simulink model "BaseEngineController_LS_128"  (Simulink 7.7)
settings: Solver=FixedStepDiscrete  StartTime=0.0  StopTime=10.0  RelTol=1e-3
PreLoadFcn:
  | try, eval([bdroot '_setup']); catch, eval('model_setup', ''); end
InitFcn:
  | try, eval([bdroot '_setup']); catch, eval('model_setup', ''); end
undefined symbols (not defined in the file): ECU565, High, motohawk_build_version, motohawk_trunc_name, motohawk_vardec_config_group, motohawk_vardec_path, True
libraries: MotoHawk_lib x1418, motohawk_control_primitives_lib x183, motohawk_engine_lib x32, simulink x21, motohawk_annotations_lib x9, AutoDoc_lib x8, simulink_extras x4, motohawk_ccp_examples_lib x1, motohawk_control_primitives_motoshare_lib x1
(part 9 of 27)

== system BaseEngineController_LS_128/Foreground/Inputs/NonLinearSensors/Temp Sensors ==
  Trigger : TriggerPort  TriggerType=function-call
  CAT1 : motohawk_engine_lib/Non-Linear Sensor Characterization (tbl)  SystemSampleTime=-1  nam='CAT'  prefix='CAT'  units='C'  inputunits='ADC'  parent_group=motohawk_vardec_path(gcb)  tblsize=13  samp_time=-1
  "ECT " : motohawk_engine_lib/Non-Linear Sensor Characterization (tbl)  SystemSampleTime=-1  nam='ECT'  prefix='ECT'  units='C'  inputunits='ADC'  parent_group=motohawk_vardec_path(gcb)  tblsize=13  samp_time=-1
  "EVAP " : motohawk_engine_lib/Non-Linear Sensor Characterization (tbl)  SystemSampleTime=-1  nam='EVAP'  prefix='EVAP'  units='C'  inputunits='ADC'  parent_group=motohawk_vardec_path(gcb)  tblsize=13  samp_time=-1
  "IAT " : motohawk_engine_lib/Non-Linear Sensor Characterization (tbl)  SystemSampleTime=-1  nam='IAT'  prefix='IAT'  units='C'  inputunits='ADC'  parent_group=motohawk_vardec_path(gcb)  tblsize=13  samp_time=-1
  motohawk_ain : MotoHawk_lib/Analog I//O Blocks/motohawk_ain  res_name=[]  text_resource=AN10M  code_resource=RES_ECUP  val_resource=-1  target=ECU565-128  resource_enum_str=(None)=-1,ECUP=53,DRVP=54,XDRP=55,AN1M=56,AN2M=57,AN3M=58,AN4M=59,AN5M=60,AN6M=61,AN7M=62,AN8M=63,AN9M=64,AN10M=65,AN11M=66,AN12M=67,AN13M=68,AN14M=69,AN15M=70,AN16M=71,AN17M=72,AN18M=73,AN19M=74,AN20M=75,AN21M=76,AN22M=77,AN23M=78,AN24M=79,AN25M=80,AN26M=81,AN27M=82,AN28M=83,AN29M=84,AN30M=85,AN31M=86,AN32M=87,AN33M=88,AN34M=89,O2A=90,O2B=91,XDRP_B=92,REF_14V=143  altref=5V Reference  typ=uint16  num_adc_bits=10  use_stat=off  use_vardec=on  nam='ECTSensorPin'  read_level=1  write_level=1  group='System | I/O Pins | Inputs Config'
  motohawk_ain1 : MotoHawk_lib/Analog I//O Blocks/motohawk_ain  res_name=[]  text_resource=AN9M  code_resource=RES_ECUP  val_resource=-1  target=ECU565-128  resource_enum_str=(None)=-1,ECUP=53,DRVP=54,XDRP=55,AN1M=56,AN2M=57,AN3M=58,AN4M=59,AN5M=60,AN6M=61,AN7M=62,AN8M=63,AN9M=64,AN10M=65,AN11M=66,AN12M=67,AN13M=68,AN14M=69,AN15M=70,AN16M=71,AN17M=72,AN18M=73,AN19M=74,AN20M=75,AN21M=76,AN22M=77,AN23M=78,AN24M=79,AN25M=80,AN26M=81,AN27M=82,AN28M=83,AN29M=84,AN30M=85,AN31M=86,AN32M=87,AN33M=88,AN34M=89,O2A=90,O2B=91,XDRP_B=92,REF_14V=143  altref=5V Reference  typ=uint16  num_adc_bits=10  use_stat=off  use_vardec=on  nam='IATSensorPin'  read_level=1  write_level=1  group='System | I/O Pins | Inputs Config'
  motohawk_ain2 : MotoHawk_lib/Analog I//O Blocks/motohawk_ain  res_name=[]  text_resource=AN11M  code_resource=RES_ECUP  val_resource=-1  target=ECU565-128  resource_enum_str=(None)=-1,ECUP=53,DRVP=54,XDRP=55,AN1M=56,AN2M=57,AN3M=58,AN4M=59,AN5M=60,AN6M=61,AN7M=62,AN8M=63,AN9M=64,AN10M=65,AN11M=66,AN12M=67,AN13M=68,AN14M=69,AN15M=70,AN16M=71,AN17M=72,AN18M=73,AN19M=74,AN20M=75,AN21M=76,AN22M=77,AN23M=78,AN24M=79,AN25M=80,AN26M=81,AN27M=82,AN28M=83,AN29M=84,AN30M=85,AN31M=86,AN32M=87,AN33M=88,AN34M=89,O2A=90,O2B=91,XDRP_B=92,REF_14V=143  altref=5V Reference  typ=uint16  num_adc_bits=10  use_stat=off  use_vardec=on  nam='EVAPSensorPin'  read_level=1  write_level=1  group='System | I/O Pins | Inputs Config'
  motohawk_ain3 : MotoHawk_lib/Analog I//O Blocks/motohawk_ain  res_name=[]  text_resource=AN12M  code_resource=RES_ECUP  val_resource=-1  target=ECU565-128  resource_enum_str=(None)=-1,ECUP=53,DRVP=54,XDRP=55,AN1M=56,AN2M=57,AN3M=58,AN4M=59,AN5M=60,AN6M=61,AN7M=62,AN8M=63,AN9M=64,AN10M=65,AN11M=66,AN12M=67,AN13M=68,AN14M=69,AN15M=70,AN16M=71,AN17M=72,AN18M=73,AN19M=74,AN20M=75,AN21M=76,AN22M=77,AN23M=78,AN24M=79,AN25M=80,AN26M=81,AN27M=82,AN28M=83,AN29M=84,AN30M=85,AN31M=86,AN32M=87,AN33M=88,AN34M=89,O2A=90,O2B=91,XDRP_B=92,REF_14V=143  altref=5V Reference  typ=uint16  num_adc_bits=10  use_stat=off  use_vardec=on  nam='CATSensorPin'  read_level=1  write_level=1  group='System | I/O Pins | Inputs Config'
  ECT : Outport
  ECT_Raw : Outport  Port=2
  IAT : Outport  Port=3
  IAT_Raw : Outport  Port=4
  EVAP : Outport  Port=5
  EVAP_Raw : Outport  Port=6
  CAT : Outport  Port=7
  CAT_Raw : Outport  Port=8
  wires:
  motohawk_ain1/1 -> "IAT "/1
  motohawk_ain/1 -> "ECT "/1
  "ECT "/1 -> ECT/1
  "ECT "/2 -> ECT_Raw/1
  "IAT "/1 -> IAT/1  "IAT"
  "IAT "/2 -> IAT_Raw/1  "IAT_Raw"
  motohawk_ain2/1 -> "EVAP "/1
  "EVAP "/1 -> EVAP/1  "IAT"
  "EVAP "/2 -> EVAP_Raw/1  "IAT_Raw"
  motohawk_ain3/1 -> CAT1/1
  CAT1/1 -> CAT/1  "IAT"
  CAT1/2 -> CAT_Raw/1  "IAT_Raw"

== system BaseEngineController_LS_128/Foreground/Inputs/PotentiometerSensors/APP1 ==
  note: Non-Linear Scaling from ADC Counts
      | to Engineering Units
  note: Faults for
      | Out-of-Range
      | Input
  ADC : Inport
  Constant1 : Constant  Value=0  OutDataTypeStr=double
  Data Type Conversion : DataTypeConversion  SaturateOnIntegerOverflow=on  RndMeth=Zero
  Final Value : MotoHawk_lib/Calibration & Probing Blocks/motohawk_probe  nam=nam  show_more=on  name_source=Use Parameter  read_level=1  view_as=Number  enum_struct={'Disabled', 'Enabled'}  vector_style=Wide Row  use_help_units=on  help='Final value after Linear Sensor Characterization'  units=units  use_header_enum=off  row_header_enum={}  col_header_enum={}  use_precision=off  precision=''  gain=1  offset=0  exp=1  use_mototune_group=on  mototune_group=group
  First Order Low Pass : motohawk_control_primitives_lib/First Order Low Pass (Tunable)  SystemSampleTime=-1  nam=[prefix 'FiltConst']  samp_time=samp_time  group=[group ' | ' nam ' Config']
  From Analog Input : MotoHawk_lib/Calibration & Probing Blocks/motohawk_probe  nam=[prefix 'ADC']  show_more=on  name_source=Use Parameter  read_level=1  view_as=Number  enum_struct={'Disabled', 'Enabled'}  vector_style=Wide Row  use_help_units=on  help='Signal measured directly from sensor'  units=inputunits  use_header_enum=off  row_header_enum={}  col_header_enum={}  use_precision=off  precision=''  gain=1  offset=0  exp=1  use_mototune_group=on  mototune_group=group
  If : If  NumInputs=2  IfExpression=u1  ElseIfExpressions=u2  ZeroCross=off
  If Action Subsystem : Subsystem  TreatAsAtomicUnit=on
      mask Display: disp('Saturate');
  If Action Subsystem1 : Subsystem  TreatAsAtomicUnit=on
      mask Display: disp('Default');
  If Action Subsystem2 : Subsystem  TreatAsAtomicUnit=on
      mask Display: disp('Pass Through');
  Logical Operator1 : Logic  Operator=OR
  Logical Operator2 : Logic
  Logical Operator3 : Logic
  Logical Operator4 : Logic  Operator=OR
  Logical Operator5 : Logic
  Logical Operator6 : Logic  Operator=NOT
  Merge : Merge  Inputs=3
  Override : MotoHawk_lib/Calibration & Probing Blocks/motohawk_override_abs  SystemSampleTime=-1  parent_name=nam  parent_val=0  show_more=on  name_source=Use Parameter  parent_read_level=1  parent_override_level=1  view_as=Number  enum_struct={'Disabled', 'Enabled'}  use_help_units=on  parent_help='Override result of linear sensor characterization, in engineering units'  parent_units=units  use_min_max=on  parent_min=-inf  parent_max=inf  use_precision=off  parent_precision=''  parent_gain=1  parent_offset=0  parent_exp=1  use_mototune_group=on  parent_group=group
  Relational Operator2 : RelationalOperator  Operator=>  ZeroCross=off  InputSameDT=on
  Relational Operator3 : RelationalOperator  Operator=<  ZeroCross=off  InputSameDT=on
  Saturation : motohawk_control_primitives_lib/Saturation  SystemSampleTime=-1
  "Unfiltered, Before Range Checking" : MotoHawk_lib/Calibration & Probing Blocks/motohawk_probe  nam=[prefix 'Raw']  show_more=on  name_source=Use Parameter  read_level=1  view_as=Number  enum_struct={'Disabled', 'Enabled'}  vector_style=Wide Row  use_help_units=on  help='After conversion to engineering units, before range checking'  units=units  use_header_enum=off  row_header_enum={}  col_header_enum={}  use_precision=off  precision=''  gain=1  offset=0  exp=1  use_mototune_group=on  mototune_group=group
  Unit Delay : UnitDelay  SampleTime=-1
  motohawk_calibration1 : MotoHawk_lib/Calibration & Probing Blocks/motohawk_calibration  nam=[prefix 'Max']  val=1020  storage=Calibration  show_more=on  name_source=Use Parameter  data_type=double  read_level=1  write_level=1  ovr_cals=on  view_as=Number  enum_struct={'Disabled', 'Enabled'}  vector_style=Wide Row  use_help_units=on  help='Maximum allowable input, indicating short or open circuit'  units=inputunits  use_header_enum=off  row_header_enum={}  col_header_enum={}  use_min_max=off  min_val=-inf  max_val=inf  use_precision=off  precision=''  gain=1  offset=0  exp=1  use_mototune_group=on  mototune_group=[group ' | ' nam ' Config']
  motohawk_calibration2 : MotoHawk_lib/Calibration & Probing Blocks/motohawk_calibration  nam=[prefix 'MaxLimit']  val=100  storage=Calibration  show_more=on  name_source=Use Parameter  data_type=double  read_level=1  write_level=1  ovr_cals=on  view_as=Number  enum_struct={'Disabled', 'Enabled'}  vector_style=Wide Row  use_help_units=on  help='Sets the upper limit on the potentiometer range.'  units=units  use_header_enum=off  row_header_enum={}  col_header_enum={}  use_min_max=off  min_val=-inf  max_val=inf  use_precision=off  precision=''  gain=1  offset=0  exp=1  use_mototune_group=on  mototune_group=[group ' | ' nam ' Config']
  motohawk_calibration3 : MotoHawk_lib/Calibration & Probing Blocks/motohawk_calibration  nam=[prefix 'Default']  val=0  storage=Calibration  show_more=on  name_source=Use Parameter  data_type=double  read_level=1  write_level=1  ovr_cals=on  view_as=Number  enum_struct={'Disabled', 'Enabled'}  vector_style=Wide Row  use_help_units=on  help="'This is the initial default value should the sensor be in fault on key-up.  Otherwise the sensors outputs the last value prior to faulting'"  units=units  use_header_enum=off  row_header_enum={}  col_header_enum={}  use_min_max=off  min_val=-inf  max_val=inf  use_precision=off  precision=''  gain=1  offset=0  exp=1  use_mototune_group=on  mototune_group=[group ' | ' nam ' Config']
  motohawk_calibration6 : MotoHawk_lib/Calibration & Probing Blocks/motohawk_calibration  nam=[prefix 'Min']  val=10  storage=Calibration  show_more=on  name_source=Use Parameter  data_type=double  read_level=1  write_level=1  ovr_cals=on  view_as=Number  enum_struct={'Disabled', 'Enabled'}  vector_style=Wide Row  use_help_units=on  help='Minimum allowable input, indicating short or open circuit'  units=inputunits  use_header_enum=off  row_header_enum={}  col_header_enum={}  use_min_max=off  min_val=-inf  max_val=inf  use_precision=off  precision=''  gain=1  offset=0  exp=1  use_mototune_group=on  mototune_group=[group ' | ' nam ' Config']
  motohawk_data_read1 : MotoHawk_lib/Data Storage Blocks/motohawk_data_read  source=Lookup By Name  structure=Scalar  operation=Read entire data structure at once  sz_vec=4  sz_row=2  sz_col=3  typ=boolean  nam='MPRD'  checkNull=on  struct_inst_name='Struct1'  struct_nam='MyStruct'
  motohawk_fault_def2 : MotoHawk_lib/Fault Management Blocks/motohawk_fault_def  nam=[prefix 'RangeHigh']  mode=Enabled  id=[]  x=25  y=50  input_suspected=on  indeterminate=off  increment_xy=on  downsample_count=1  ovr_cals=on  ovr_actions=on  show_actions=off  action1_name=''  action1_cond=(None)  action2_name=''  action2_cond=(None)  action3_name=''  action3_cond=(None)  action4_name=''  action4_cond=(None)
  motohawk_fault_def3 : MotoHawk_lib/Fault Management Blocks/motohawk_fault_def  nam=[prefix 'RangeLow']  mode=Enabled  id=[]  x=25  y=50  input_suspected=on  indeterminate=off  increment_xy=on  downsample_count=1  ovr_cals=on  ovr_actions=on  show_actions=off  action1_name=''  action1_cond=(None)  action2_name=''  action2_cond=(None)  action3_name=''  action3_cond=(None)  action4_name=''  action4_cond=(None)
  motohawk_fault_status1 : MotoHawk_lib/Fault Management Blocks/motohawk_fault_status  source=Lookup By Name  nam=[prefix 'RangeHigh']  status=Active
  motohawk_fault_status2 : MotoHawk_lib/Fault Management Blocks/motohawk_fault_status  source=Lookup By Name  nam=[prefix 'RangeHigh']  status=Suspected
  motohawk_fault_status3 : MotoHawk_lib/Fault Management Blocks/motohawk_fault_status  source=Lookup By Name  nam=[prefix 'RangeLow']  status=Suspected
  motohawk_fault_status4 : MotoHawk_lib/Fault Management Blocks/motohawk_fault_status  source=Lookup By Name  nam=[prefix 'RangeLow']  status=Active
  motohawk_table_1d1 : MotoHawk_lib/Lookup Tables/motohawk_table_1d  SystemSampleTime=-1  nam=nam  bp_nam=''  breakpoint_data=[1:tblsize]  table_data=[1:tblsize]  show_more=on  bp_data_type=Inherit from 'Breakpoint Data'  bp_storage=Constant  table_data_type=Inherit from 'Table Data'  storage=NonAdaptive  read_level=1  write_level=1  ovr_cals=on  use_help=on  help='Look up table to allownon-linear characterization of sensors'  bp_units=inputunits  table_units=units  use_min_max=off  bp_min_val=-inf  bp_max_val=inf  min_val=-inf  max_val=inf  use_precision=off  use_breakpoint=off  b_precision=''  b_gain=1  b_offset=0  b_exp=1  use_table=off  t_precision=''  t_gain=1  t_offset=0  t_exp=1  use_links=off  input_name=[prefix 'ADC']  output_name=[prefix 'Raw']  use_mototune_group=on  mototune_group=group
  EngUnitsFilt : Outport
  EngUnitsRaw : Outport  Port=2
  wires:
  Logical Operator5/1 -> If/1
  Logical Operator1/1 -> Logical Operator5/2
  Logical Operator4/1 -> If/2, Logical Operator6/1
  Logical Operator6/1 -> Logical Operator5/1
  First Order Low Pass/1 -> Override/1
  motohawk_calibration3/1 -> If Action Subsystem1/1(In)
  If Action Subsystem1/1(Out) -> Merge/3
  If/2 -> If Action Subsystem1/Action
  motohawk_fault_status4/1 -> Logical Operator4/2
  motohawk_fault_status1/1 -> Logical Operator4/1
  ADC/1 -> From Analog Input/1, Data Type Conversion/1
  Unit Delay/1 -> If Action Subsystem/1(In)
  motohawk_table_1d1/1 -> "Unfiltered, Before Range Checking"/1, If Action Subsystem2/1(In)
  If Action Subsystem/1(Out) -> Merge/2
  If Action Subsystem2/1(Out) -> Merge/1
  motohawk_fault_status3/1 -> Logical Operator1/2
  motohawk_fault_status2/1 -> Logical Operator1/1
  motohawk_calibration6/1 -> Relational Operator3/2
  motohawk_calibration1/1 -> Relational Operator2/2
  Relational Operator2/1 -> Logical Operator2/2
  Relational Operator3/1 -> Logical Operator3/2
  Logical Operator2/1 -> motohawk_fault_def2/1
  Logical Operator3/1 -> motohawk_fault_def3/1
  motohawk_data_read1/1 -> Logical Operator3/1, Logical Operator2/1
  Override/1 -> EngUnitsFilt/1, Final Value/1
  Data Type Conversion/1 -> motohawk_table_1d1/1, Relational Operator3/1, Relational Operator2/1
  If/1 -> If Action Subsystem/Action
  If/3 -> If Action Subsystem2/Action
  motohawk_calibration2/1 -> Saturation/3
  Constant1/1 -> Saturation/2
  Merge/1 -> Saturation/1
  Saturation/1 -> Unit Delay/1, EngUnitsRaw/1, First Order Low Pass/1

== system BaseEngineController_LS_128/Foreground/Inputs/PotentiometerSensors/APP1ForcedAdapt ==
  Documentation_Calibrations_Probes_Block : AutoDoc_lib/Documentation_Calibrations_Probes_Block
  Function-Call Subsystem : Subsystem  TreatAsAtomicUnit=on
  Logical Operator : Logic  AllPortsSameDT=off  OutDataTypeStr=boolean
  Logical Operator1 : Logic  AllPortsSameDT=off  OutDataTypeStr=boolean
  Relational Operator : RelationalOperator  Operator=<  OutDataTypeStr=boolean
  Relational Operator1 : RelationalOperator  Operator=>  OutDataTypeStr=boolean
  motohawk_calibration : MotoHawk_lib/Calibration & Probing Blocks/motohawk_calibration  nam='APP1LowAdaptADCThresh'  val=300  storage=Calibration  show_more=on  name_source=Use Parameter  data_type=Inherit from 'Default Value'  read_level=1  write_level=1  ovr_cals=on  view_as=Number  enum_struct={'Disabled', 'Enabled'}  vector_style=Wide Row  use_help_units=on  help='Sets the ADC limit below which a low-side adapt will be captured on key-up.'  units='ADC'  use_header_enum=off  row_header_enum={}  col_header_enum={}  use_min_max=off  min_val=-inf  max_val=inf  use_precision=off  precision=''  gain=1  offset=0  exp=1  use_mototune_group=on  mototune_group=motohawk_vardec_path(gcb)
  motohawk_calibration1 : MotoHawk_lib/Calibration & Probing Blocks/motohawk_calibration  nam='APP1HiAdaptADCThresh'  val=700  storage=Calibration  show_more=on  name_source=Use Parameter  data_type=Inherit from 'Default Value'  read_level=1  write_level=1  ovr_cals=on  view_as=Number  enum_struct={'Disabled', 'Enabled'}  vector_style=Wide Row  use_help_units=on  help='Sets the ADC limit above which a high-side adapt will be captured on key-up.'  units='ADC'  use_header_enum=off  row_header_enum={}  col_header_enum={}  use_min_max=off  min_val=-inf  max_val=inf  use_precision=off  precision=''  gain=1  offset=0  exp=1  use_mototune_group=on  mototune_group=motohawk_vardec_path(gcb)
  motohawk_data_read1 : MotoHawk_lib/Data Storage Blocks/motohawk_data_read  source=Lookup By Name  structure=Scalar  operation=Read scalar from location by index  sz_vec=4  sz_row=2  sz_col=3  typ=double  nam='APP1_AdaptADC'  checkNull=on  struct_inst_name='Struct1'  struct_nam='MyStruct'
  motohawk_trigger : MotoHawk_lib/Trigger Blocks/motohawk_trigger  Tag=Trigger  trigger=FGND_20XRTI_PERIODIC  function_name=Trigger_FGND_20XRTI_PERIODIC_9951p0004  priority_order=0  inherited=on  run_disabled=off  override_app_monitor=off  target=ECU565_128
  LowSide Request : Outport
  HiSide Request : Outport  Port=2
  wires:
  motohawk_trigger/1 -> Function-Call Subsystem/Trigger
  Function-Call Subsystem/1(Out1) -> Logical Operator/1, Logical Operator1/1
  motohawk_data_read1/1 -> Relational Operator/1, Relational Operator1/1
  Relational Operator/1 -> Logical Operator/2
  motohawk_calibration/1 -> Relational Operator/2
  motohawk_calibration1/1 -> Relational Operator1/2
  Relational Operator1/1 -> Logical Operator1/2
  Logical Operator/1 -> LowSide Request/1
  Logical Operator1/1 -> HiSide Request/1

== system BaseEngineController_LS_128/Foreground/Inputs/PotentiometerSensors/APP2 ==
  note: Non-Linear Scaling from ADC Counts
      | to Engineering Units
  note: Faults for
      | Out-of-Range
      | Input
  ADC : Inport
  Constant1 : Constant  Value=0  OutDataTypeStr=double
  Data Type Conversion : DataTypeConversion  SaturateOnIntegerOverflow=on  RndMeth=Zero
  Final Value : MotoHawk_lib/Calibration & Probing Blocks/motohawk_probe  nam=nam  show_more=on  name_source=Use Parameter  read_level=1  view_as=Number  enum_struct={'Disabled', 'Enabled'}  vector_style=Wide Row  use_help_units=on  help='Final value after Linear Sensor Characterization'  units=units  use_header_enum=off  row_header_enum={}  col_header_enum={}  use_precision=off  precision=''  gain=1  offset=0  exp=1  use_mototune_group=on  mototune_group=group
  First Order Low Pass : motohawk_control_primitives_lib/First Order Low Pass (Tunable)  SystemSampleTime=-1  nam=[prefix 'FiltConst']  samp_time=samp_time  group=[group ' | ' nam ' Config']
  From Analog Input : MotoHawk_lib/Calibration & Probing Blocks/motohawk_probe  nam=[prefix 'ADC']  show_more=on  name_source=Use Parameter  read_level=1  view_as=Number  enum_struct={'Disabled', 'Enabled'}  vector_style=Wide Row  use_help_units=on  help='Signal measured directly from sensor'  units=inputunits  use_header_enum=off  row_header_enum={}  col_header_enum={}  use_precision=off  precision=''  gain=1  offset=0  exp=1  use_mototune_group=on  mototune_group=group
  If : If  NumInputs=2  IfExpression=u1  ElseIfExpressions=u2  ZeroCross=off
  If Action Subsystem : Subsystem  TreatAsAtomicUnit=on
      mask Display: disp('Saturate');
  If Action Subsystem1 : Subsystem  TreatAsAtomicUnit=on
      mask Display: disp('Default');
  If Action Subsystem2 : Subsystem  TreatAsAtomicUnit=on
      mask Display: disp('Pass Through');
  Logical Operator1 : Logic  Operator=OR
  Logical Operator2 : Logic
  Logical Operator3 : Logic
  Logical Operator4 : Logic  Operator=OR
  Logical Operator5 : Logic
  Logical Operator6 : Logic  Operator=NOT
  Merge : Merge  Inputs=3
  Override : MotoHawk_lib/Calibration & Probing Blocks/motohawk_override_abs  SystemSampleTime=-1  parent_name=nam  parent_val=0  show_more=on  name_source=Use Parameter  parent_read_level=1  parent_override_level=1  view_as=Number  enum_struct={'Disabled', 'Enabled'}  use_help_units=on  parent_help='Override result of linear sensor characterization, in engineering units'  parent_units=units  use_min_max=on  parent_min=-inf  parent_max=inf  use_precision=off  parent_precision=''  parent_gain=1  parent_offset=0  parent_exp=1  use_mototune_group=on  parent_group=group
  Relational Operator2 : RelationalOperator  Operator=>  ZeroCross=off  InputSameDT=on
  Relational Operator3 : RelationalOperator  Operator=<  ZeroCross=off  InputSameDT=on
  Saturation : motohawk_control_primitives_lib/Saturation  SystemSampleTime=-1
  "Unfiltered, Before Range Checking" : MotoHawk_lib/Calibration & Probing Blocks/motohawk_probe  nam=[prefix 'Raw']  show_more=on  name_source=Use Parameter  read_level=1  view_as=Number  enum_struct={'Disabled', 'Enabled'}  vector_style=Wide Row  use_help_units=on  help='After conversion to engineering units, before range checking'  units=units  use_header_enum=off  row_header_enum={}  col_header_enum={}  use_precision=off  precision=''  gain=1  offset=0  exp=1  use_mototune_group=on  mototune_group=group
  Unit Delay : UnitDelay  SampleTime=-1
  motohawk_calibration1 : MotoHawk_lib/Calibration & Probing Blocks/motohawk_calibration  nam=[prefix 'Max']  val=1020  storage=Calibration  show_more=on  name_source=Use Parameter  data_type=double  read_level=1  write_level=1  ovr_cals=on  view_as=Number  enum_struct={'Disabled', 'Enabled'}  vector_style=Wide Row  use_help_units=on  help='Maximum allowable input, indicating short or open circuit'  units=inputunits  use_header_enum=off  row_header_enum={}  col_header_enum={}  use_min_max=off  min_val=-inf  max_val=inf  use_precision=off  precision=''  gain=1  offset=0  exp=1  use_mototune_group=on  mototune_group=[group ' | ' nam ' Config']
  motohawk_calibration2 : MotoHawk_lib/Calibration & Probing Blocks/motohawk_calibration  nam=[prefix 'MaxLimit']  val=100  storage=Calibration  show_more=on  name_source=Use Parameter  data_type=double  read_level=1  write_level=1  ovr_cals=on  view_as=Number  enum_struct={'Disabled', 'Enabled'}  vector_style=Wide Row  use_help_units=on  help='Sets the upper limit on the potentiometer range.'  units=units  use_header_enum=off  row_header_enum={}  col_header_enum={}  use_min_max=off  min_val=-inf  max_val=inf  use_precision=off  precision=''  gain=1  offset=0  exp=1  use_mototune_group=on  mototune_group=[group ' | ' nam ' Config']
  motohawk_calibration3 : MotoHawk_lib/Calibration & Probing Blocks/motohawk_calibration  nam=[prefix 'Default']  val=0  storage=Calibration  show_more=on  name_source=Use Parameter  data_type=double  read_level=1  write_level=1  ovr_cals=on  view_as=Number  enum_struct={'Disabled', 'Enabled'}  vector_style=Wide Row  use_help_units=on  help="'This is the initial default value should the sensor be in fault on key-up.  Otherwise the sensors outputs the last value prior to faulting'"  units=units  use_header_enum=off  row_header_enum={}  col_header_enum={}  use_min_max=off  min_val=-inf  max_val=inf  use_precision=off  precision=''  gain=1  offset=0  exp=1  use_mototune_group=on  mototune_group=[group ' | ' nam ' Config']
  motohawk_calibration6 : MotoHawk_lib/Calibration & Probing Blocks/motohawk_calibration  nam=[prefix 'Min']  val=10  storage=Calibration  show_more=on  name_source=Use Parameter  data_type=double  read_level=1  write_level=1  ovr_cals=on  view_as=Number  enum_struct={'Disabled', 'Enabled'}  vector_style=Wide Row  use_help_units=on  help='Minimum allowable input, indicating short or open circuit'  units=inputunits  use_header_enum=off  row_header_enum={}  col_header_enum={}  use_min_max=off  min_val=-inf  max_val=inf  use_precision=off  precision=''  gain=1  offset=0  exp=1  use_mototune_group=on  mototune_group=[group ' | ' nam ' Config']
  motohawk_data_read1 : MotoHawk_lib/Data Storage Blocks/motohawk_data_read  source=Lookup By Name  structure=Scalar  operation=Read entire data structure at once  sz_vec=4  sz_row=2  sz_col=3  typ=boolean  nam='MPRD'  checkNull=on  struct_inst_name='Struct1'  struct_nam='MyStruct'
  motohawk_fault_def2 : MotoHawk_lib/Fault Management Blocks/motohawk_fault_def  nam=[prefix 'RangeHigh']  mode=Enabled  id=[]  x=25  y=50  input_suspected=on  indeterminate=off  increment_xy=on  downsample_count=1  ovr_cals=on  ovr_actions=on  show_actions=off  action1_name=''  action1_cond=(None)  action2_name=''  action2_cond=(None)  action3_name=''  action3_cond=(None)  action4_name=''  action4_cond=(None)
  motohawk_fault_def3 : MotoHawk_lib/Fault Management Blocks/motohawk_fault_def  nam=[prefix 'RangeLow']  mode=Enabled  id=[]  x=25  y=50  input_suspected=on  indeterminate=off  increment_xy=on  downsample_count=1  ovr_cals=on  ovr_actions=on  show_actions=off  action1_name=''  action1_cond=(None)  action2_name=''  action2_cond=(None)  action3_name=''  action3_cond=(None)  action4_name=''  action4_cond=(None)
  motohawk_fault_status1 : MotoHawk_lib/Fault Management Blocks/motohawk_fault_status  source=Lookup By Name  nam=[prefix 'RangeHigh']  status=Active
  motohawk_fault_status2 : MotoHawk_lib/Fault Management Blocks/motohawk_fault_status  source=Lookup By Name  nam=[prefix 'RangeHigh']  status=Suspected
  motohawk_fault_status3 : MotoHawk_lib/Fault Management Blocks/motohawk_fault_status  source=Lookup By Name  nam=[prefix 'RangeLow']  status=Suspected
  motohawk_fault_status4 : MotoHawk_lib/Fault Management Blocks/motohawk_fault_status  source=Lookup By Name  nam=[prefix 'RangeLow']  status=Active
  motohawk_table_1d1 : MotoHawk_lib/Lookup Tables/motohawk_table_1d  SystemSampleTime=-1  nam=nam  bp_nam=''  breakpoint_data=[1:tblsize]  table_data=[1:tblsize]  show_more=on  bp_data_type=Inherit from 'Breakpoint Data'  bp_storage=Constant  table_data_type=Inherit from 'Table Data'  storage=NonAdaptive  read_level=1  write_level=1  ovr_cals=on  use_help=on  help='Look up table to allownon-linear characterization of sensors'  bp_units=inputunits  table_units=units  use_min_max=off  bp_min_val=-inf  bp_max_val=inf  min_val=-inf  max_val=inf  use_precision=off  use_breakpoint=off  b_precision=''  b_gain=1  b_offset=0  b_exp=1  use_table=off  t_precision=''  t_gain=1  t_offset=0  t_exp=1  use_links=off  input_name=[prefix 'ADC']  output_name=[prefix 'Raw']  use_mototune_group=on  mototune_group=group
  EngUnitsFilt : Outport
  EngUnitsRaw : Outport  Port=2
  wires:
  Logical Operator5/1 -> If/1
  Logical Operator1/1 -> Logical Operator5/2
  Logical Operator4/1 -> If/2, Logical Operator6/1
  Logical Operator6/1 -> Logical Operator5/1
  First Order Low Pass/1 -> Override/1
  motohawk_calibration3/1 -> If Action Subsystem1/1(In)
  If Action Subsystem1/1(Out) -> Merge/3
  If/2 -> If Action Subsystem1/Action
  motohawk_fault_status4/1 -> Logical Operator4/2
  motohawk_fault_status1/1 -> Logical Operator4/1
  ADC/1 -> From Analog Input/1, Data Type Conversion/1
  Unit Delay/1 -> If Action Subsystem/1(In)
  motohawk_table_1d1/1 -> "Unfiltered, Before Range Checking"/1, If Action Subsystem2/1(In)
  If Action Subsystem/1(Out) -> Merge/2
  If Action Subsystem2/1(Out) -> Merge/1
  motohawk_fault_status3/1 -> Logical Operator1/2
  motohawk_fault_status2/1 -> Logical Operator1/1
  motohawk_calibration6/1 -> Relational Operator3/2
  motohawk_calibration1/1 -> Relational Operator2/2
  Relational Operator2/1 -> Logical Operator2/2
  Relational Operator3/1 -> Logical Operator3/2
  Logical Operator2/1 -> motohawk_fault_def2/1
  Logical Operator3/1 -> motohawk_fault_def3/1
  motohawk_data_read1/1 -> Logical Operator3/1, Logical Operator2/1
  Override/1 -> EngUnitsFilt/1, Final Value/1
  Data Type Conversion/1 -> motohawk_table_1d1/1, Relational Operator3/1, Relational Operator2/1
  If/1 -> If Action Subsystem/Action
  If/3 -> If Action Subsystem2/Action
  motohawk_calibration2/1 -> Saturation/3
  Constant1/1 -> Saturation/2
  Merge/1 -> Saturation/1
  Saturation/1 -> Unit Delay/1, EngUnitsRaw/1, First Order Low Pass/1

== system BaseEngineController_LS_128/Foreground/Inputs/PotentiometerSensors/APP2ForcedAdapt ==
  Function-Call Subsystem : Subsystem  TreatAsAtomicUnit=on
  Logical Operator : Logic  AllPortsSameDT=off  OutDataTypeStr=boolean
  Logical Operator1 : Logic  AllPortsSameDT=off  OutDataTypeStr=boolean
  Relational Operator : RelationalOperator  Operator=<  OutDataTypeStr=boolean
  Relational Operator1 : RelationalOperator  Operator=>  OutDataTypeStr=boolean
  motohawk_calibration : MotoHawk_lib/Calibration & Probing Blocks/motohawk_calibration  nam='APP2LowAdaptADCThresh'  val=300  storage=Calibration  show_more=on  name_source=Use Parameter  data_type=Inherit from 'Default Value'  read_level=1  write_level=1  ovr_cals=on  view_as=Number  enum_struct={'Disabled', 'Enabled'}  vector_style=Wide Row  use_help_units=on  help='Sets the ADC limit below which a low-side adapt will be captured on key-up.'  units='ADC'  use_header_enum=off  row_header_enum={}  col_header_enum={}  use_min_max=off  min_val=-inf  max_val=inf  use_precision=off  precision=''  gain=1  offset=0  exp=1  use_mototune_group=on  mototune_group=motohawk_vardec_path(gcb)
  motohawk_calibration1 : MotoHawk_lib/Calibration & Probing Blocks/motohawk_calibration  nam='APP2HiAdaptADCThresh'  val=700  storage=Calibration  show_more=on  name_source=Use Parameter  data_type=Inherit from 'Default Value'  read_level=1  write_level=1  ovr_cals=on  view_as=Number  enum_struct={'Disabled', 'Enabled'}  vector_style=Wide Row  use_help_units=on  help='Sets the ADC limit above which a high-side adapt will be captured on key-up.'  units='ADC'  use_header_enum=off  row_header_enum={}  col_header_enum={}  use_min_max=off  min_val=-inf  max_val=inf  use_precision=off  precision=''  gain=1  offset=0  exp=1  use_mototune_group=on  mototune_group=motohawk_vardec_path(gcb)
  motohawk_data_read1 : MotoHawk_lib/Data Storage Blocks/motohawk_data_read  source=Lookup By Name  structure=Scalar  operation=Read scalar from location by index  sz_vec=4  sz_row=2  sz_col=3  typ=double  nam='APP2_AdaptADC'  checkNull=on  struct_inst_name='Struct1'  struct_nam='MyStruct'
  motohawk_trigger : MotoHawk_lib/Trigger Blocks/motohawk_trigger  Tag=Trigger  trigger=FGND_20XRTI_PERIODIC  function_name=Trigger_FGND_20XRTI_PERIODIC_10085p0004  priority_order=0  inherited=on  run_disabled=off  override_app_monitor=off  target=ECU565_128
  LowSide Request : Outport
  HiSide Request : Outport  Port=2
  wires:
  motohawk_trigger/1 -> Function-Call Subsystem/Trigger
  motohawk_data_read1/1 -> Relational Operator/1, Relational Operator1/1
  Relational Operator/1 -> Logical Operator/2
  motohawk_calibration/1 -> Relational Operator/2
  motohawk_calibration1/1 -> Relational Operator1/2
  Relational Operator1/1 -> Logical Operator1/2
  Logical Operator/1 -> LowSide Request/1
  Logical Operator1/1 -> HiSide Request/1
  Function-Call Subsystem/1(Out1) -> Logical Operator/1, Logical Operator1/1

== system BaseEngineController_LS_128/Foreground/Outputs/AEM Infinity Dash/Dash Custom 1 ==
  Data : Inport
  Bus Selector : BusSelector  OutputSignals=Sensors.FuelLvl_Fin
  Send CAN Messages : MotoHawk_lib/CAN Blocks/Send CAN Messages  bus=-2  nam='CAN_1'  msgl=CANTx_CUSTOM_DASH_1  pace=5  labelwires=off
  wires:
  Data/1 -> Bus Selector/1
  Bus Selector/1 -> Send CAN Messages/1  "<FuelLvl_Fin>"

== system BaseEngineController_LS_128/Foreground/Outputs/AEM Infinity Dash/Dash Message 1 ==
  Data : Inport
  Bus Selector : BusSelector  OutputSignals=Sensors.Raw.RPM,Sensors.RawProcessed.TPS,Sensors.Raw.NonLinearSensors.IAT,Sensors.Raw.NonLinearSensors.ECT
  First Order Low Pass (Tunable) : motohawk_control_primitives_lib/First Order Low Pass (Tunable)  SystemSampleTime=-1  nam='TPS_Filt'  samp_time=-1  group=motohawk_vardec_path(gcb)
  RPM_Filt : Subsystem
  Send CAN Messages : MotoHawk_lib/CAN Blocks/Send CAN Messages  bus=-2  nam='CAN_1'  msgl=CANTx_AEM_DASH_1  pace=5  labelwires=off
  wires:
  Data/1 -> Bus Selector/1
  Bus Selector/1 -> RPM_Filt/1(Raw)  "<RPM>"
  Bus Selector/2 -> First Order Low Pass (Tunable)/1  "<TPS>"
  Bus Selector/3 -> Send CAN Messages/3  "<IAT>"
  RPM_Filt/1(Filt) -> Send CAN Messages/1
  First Order Low Pass (Tunable)/1 -> Send CAN Messages/2
  Bus Selector/4 -> Send CAN Messages/4  "<ECT>"

== system BaseEngineController_LS_128/Foreground/Outputs/AEM Infinity Dash/Dash Message 2 ==
  Data : Inport
  Bus Selector : BusSelector  OutputSignals=Sensors.RawProcessed.VSPD_Final,Sensors.RawProcessed.GearEst,Controller.SparkAdv,Sensors.Raw.LinearSensors.SysVolt
  Bus Selector1 : BusSelector  OutputSignals=Sensors.Raw.CAN.O2_BankA,Sensors.Raw.CAN.O2_BUS.BANK1.DataValidState
  Bus Selector2 : BusSelector  OutputSignals=Sensors.Raw.CAN.O2_BankB,Sensors.Raw.CAN.O2_BUS.BANK2.DataValidState
  First Order Low Pass (Tunable) : motohawk_control_primitives_lib/First Order Low Pass (Tunable)  SystemSampleTime=-1  nam='VSPD_Filt'  samp_time=-1  group=motohawk_vardec_path(gcb)
  First Order Low Pass (Tunable)1 : motohawk_control_primitives_lib/First Order Low Pass (Tunable)  SystemSampleTime=-1  nam='SparkAdv_Filt'  samp_time=-1  group=motohawk_vardec_path(gcb)
  First Order Low Pass (Tunable)2 : motohawk_control_primitives_lib/First Order Low Pass (Tunable)  SystemSampleTime=-1  nam='ECUVolt_Filt'  samp_time=-1  group=motohawk_vardec_path(gcb)
  Gain : Gain  Gain=1.60934
  PHI_Filt : Subsystem
  PHI_Filt1 : Subsystem
  Send CAN Messages : MotoHawk_lib/CAN Blocks/Send CAN Messages  bus=-2  nam='CAN_1'  msgl=CANTx_AEM_DASH_2  pace=5  labelwires=off
  wires:
  Data/1 -> Bus Selector/1, Bus Selector1/1, Bus Selector2/1
  Gain/1 -> Send CAN Messages/3
  First Order Low Pass (Tunable)/1 -> Gain/1
  First Order Low Pass (Tunable)1/1 -> Send CAN Messages/5
  First Order Low Pass (Tunable)2/1 -> Send CAN Messages/6
  PHI_Filt1/1(Filt Out) -> Send CAN Messages/2
  PHI_Filt/1(Filt Out) -> Send CAN Messages/1
  Bus Selector/1 -> First Order Low Pass (Tunable)/1  "<VSPD_Final>"
  Bus Selector/2 -> Send CAN Messages/4  "<GearEst>"
  Bus Selector/3 -> First Order Low Pass (Tunable)1/1  "<SparkAdv>"
  Bus Selector/4 -> First Order Low Pass (Tunable)2/1  "<SysVolt>"
  Bus Selector1/1 -> PHI_Filt/1(PHI RAW)  "<O2_BankA>"
  Bus Selector1/2 -> PHI_Filt/2(PHI DR)  "<DataValidState>"
  Bus Selector2/1 -> PHI_Filt1/1(PHI RAW)  "<O2_BankB>"
  Bus Selector2/2 -> PHI_Filt1/2(PHI DR)  "<DataValidState>"

== system BaseEngineController_LS_128/Foreground/Outputs/AEM Infinity Dash/Dash Message 3 ==
  Data : Inport
  " " : simulink/Logic and Bit Operations/Compare To Constant  SystemSampleTime=-1  relop=>=  const=1  LogicOutDataTypeMode=uint8
  "  " : simulink/Logic and Bit Operations/Compare To Constant  SystemSampleTime=-1  relop=>=  const=1  LogicOutDataTypeMode=uint8
  "    " : Sum  Inputs=+
  "      " : Sum  Inputs=+
  " 1" : simulink/Logic and Bit Operations/Compare To Constant  SystemSampleTime=-1  relop=>=  const=3  LogicOutDataTypeMode=uint8
  Bus Selector : BusSelector  OutputSignals=Sensors.Raw.LinearSensors.MAP_Angular
  Bus Selector1 : BusSelector  OutputSignals=Sensors.Raw.LinearSensors.FuelPres,Sensors.Raw.LinearSensors.OilPres
  Bus Selector2 : BusSelector  OutputSignals=Controller.FUELP,Controller.FAN-1,Controller.FAN-2
  Bus Selector3 : BusSelector  OutputSignals=ActuatorCharacterization.FuelCutSeq,ActuatorCharacterization.SparkCutSeq
  Bus Selector4 : BusSelector  OutputSignals=Controller.AC
  Constant : Constant  Value=0
  Constant1 : Constant  Value=0
  First Order Low Pass (Tunable) : motohawk_control_primitives_lib/First Order Low Pass (Tunable)  SystemSampleTime=-1  nam='MAP_filt'  samp_time=-1  group=motohawk_vardec_path(gcb)
  First Order Low Pass (Tunable)1 : motohawk_control_primitives_lib/First Order Low Pass (Tunable)  SystemSampleTime=-1  nam='FuelPres_Filt'  samp_time=-1  group=motohawk_vardec_path(gcb)
  First Order Low Pass (Tunable)2 : motohawk_control_primitives_lib/First Order Low Pass (Tunable)  SystemSampleTime=-1  nam='OilPres_Filt'  samp_time=-1  group=motohawk_vardec_path(gcb)
  Gain : Gain  Gain=0.01
  Gain1 : Gain  Gain=0.068948
  Math Function : Math  Operator=reciprocal  SaturateOnIntegerOverflow=on
  Saturation : Saturate  UpperLimit=inf  LowerLimit=0.01
  Send CAN Messages : MotoHawk_lib/CAN Blocks/Send CAN Messages  bus=-2  nam='CAN_1'  msgl=CANTx_AEM_DASH_3  pace=5  labelwires=off
  motohawk_data_read : MotoHawk_lib/Data Storage Blocks/motohawk_data_read  source=Lookup By Name  structure=Scalar  operation=Read scalar from location by index  sz_vec=4  sz_row=2  sz_col=3  typ=double  nam='VEFin'  checkNull=on  struct_inst_name='MyData'  struct_nam='MyStruct'
  motohawk_data_read1 : MotoHawk_lib/Data Storage Blocks/motohawk_data_read  source=Lookup By Name  structure=Scalar  operation=Read scalar from location by index  sz_vec=4  sz_row=2  sz_col=3  typ=double  nam='BaseEquivRatio'  checkNull=on  struct_inst_name='MyData'  struct_nam='MyStruct'
  motohawk_data_read2 : MotoHawk_lib/Data Storage Blocks/motohawk_data_read  source=Lookup By Name  structure=Scalar  operation=Read scalar from location by index  sz_vec=4  sz_row=2  sz_col=3  typ=boolean  nam='O2CtrlMode'  checkNull=on  struct_inst_name='MyData'  struct_nam='MyStruct'
  motohawk_data_read3 : MotoHawk_lib/Data Storage Blocks/motohawk_data_read  source=Lookup By Name  structure=Scalar  operation=Read scalar from location by index  sz_vec=4  sz_row=2  sz_col=3  typ=uint8  nam='EncoderState'  checkNull=on  struct_inst_name='MyData'  struct_nam='MyStruct'
  motohawk_fault_action : MotoHawk_lib/Fault Management Blocks/motohawk_fault_action  nam='EngineProtectLED'  output_status=on  eval_nam=EngineProtectLED
  motohawk_fault_action1 : MotoHawk_lib/Fault Management Blocks/motohawk_fault_action  nam='MIL_LED'  output_status=on  eval_nam=MIL_LED
  motohawk_fault_status1 : MotoHawk_lib/Fault Management Blocks/motohawk_fault_status  source=Lookup By Name  nam='NoOil_Fault'  status=Active
  motohawk_fault_status2 : MotoHawk_lib/Fault Management Blocks/motohawk_fault_status  source=Lookup By Name  nam='LeanProtect_Fault'  status=Active
  motohawk_fault_status3 : MotoHawk_lib/Fault Management Blocks/motohawk_fault_status  source=Lookup By Name  nam='SoftOverBoost_Fault'  status=Active
  motohawk_fault_status4 : MotoHawk_lib/Fault Management Blocks/motohawk_fault_status  source=Lookup By Name  nam='ECTOverTempFault'  status=Active
  wires:
  Data/1 -> Bus Selector/1, Bus Selector1/1, Bus Selector2/1, Bus Selector4/1, Bus Selector3/1
  Bus Selector/1 -> First Order Low Pass (Tunable)/1  "<MAP_Angular>"
  motohawk_data_read/1 -> Send CAN Messages/2
  Bus Selector1/1 -> Gain/1  "<FuelPres>"
  motohawk_data_read1/1 -> Saturation/1
  Bus Selector2/3 -> Send CAN Messages/8  "<FAN-2>"
  Bus Selector2/2 -> Send CAN Messages/7  "<FAN-1>"
  Bus Selector2/1 -> Send CAN Messages/6  "<FUELP>"
  Constant/1 -> Send CAN Messages/9
  motohawk_data_read2/1 -> Send CAN Messages/10
  motohawk_fault_action/1 -> Send CAN Messages/11
  motohawk_fault_action1/1 -> Send CAN Messages/12
  motohawk_fault_status2/1 -> Send CAN Messages/13
  Math Function/1 -> Send CAN Messages/5
  motohawk_fault_status1/1 -> Send CAN Messages/14
  Bus Selector3/1 -> "    "/1  "<FuelCutSeq>"
  Bus Selector3/2 -> "      "/1  "<SparkCutSeq>"
  "    "/1 -> " "/1
  " "/1 -> Send CAN Messages/15
  "      "/1 -> "  "/1
  "  "/1 -> Send CAN Messages/16
  motohawk_data_read3/1 -> " 1"/1
  " 1"/1 -> Send CAN Messages/17
  Bus Selector4/1 -> Send CAN Messages/18  "<AC>"
  motohawk_fault_status3/1 -> Send CAN Messages/19
  motohawk_fault_status4/1 -> Send CAN Messages/20
  Constant1/1 -> Send CAN Messages/21
  Saturation/1 -> Math Function/1
  Gain/1 -> First Order Low Pass (Tunable)1/1
  Bus Selector1/2 -> Gain1/1  "<OilPres>"
  Gain1/1 -> First Order Low Pass (Tunable)2/1
  First Order Low Pass (Tunable)/1 -> Send CAN Messages/1
  First Order Low Pass (Tunable)1/1 -> Send CAN Messages/3
  First Order Low Pass (Tunable)2/1 -> Send CAN Messages/4

== system BaseEngineController_LS_128/Foreground/Outputs/AEM Infinity Dash/Dash Message 4 ==
  Data : Inport
  Bus Selector : BusSelector  OutputSignals=Sensors.AirCalcs.MAFPort,Sensors.Raw.RPM
  Bus Selector1 : BusSelector  OutputSignals=Sensors.Raw.Digital.ClutchSw
  Constant{,2..5} (5 alike) : Constant  Value=0
  Constant1 : Constant  Value=60
  Product : Product  Inputs=**/  RndMeth=Zero
  Saturation : Saturate  UpperLimit=inf  LowerLimit=.01
  Send CAN Messages : MotoHawk_lib/CAN Blocks/Send CAN Messages  bus=-2  nam='CAN_1'  msgl=CANTx_AEM_DASH_4  pace=5  labelwires=off
  wires:
  Data/1 -> Bus Selector/1, Bus Selector1/1
  Constant/1 -> Send CAN Messages/1
  Bus Selector/1 -> Send CAN Messages/2, Product/1  "<MAFPort>"
  Product/1 -> Send CAN Messages/3
  Constant1/1 -> Product/2
  Constant2/1 -> Send CAN Messages/4
  Constant3/1 -> Send CAN Messages/5
  Bus Selector1/1 -> Send CAN Messages/6  "<ClutchSw>"
  Constant4/1 -> Send CAN Messages/7
  Constant5/1 -> Send CAN Messages/8
  Saturation/1 -> Product/3
  Bus Selector/2 -> Saturation/1  "<RPM>"

== system BaseEngineController_LS_128/Foreground/Outputs/AEM Infinity Dash/Dash Message 5 ==
  Data : Inport
  Bus Selector : BusSelector  OutputSignals=Sensors.Raw.CAN.O2_BUS.BANK1.Lambda
  Constant{,1..3} (4 alike) : Constant  Value=0
  Constant4 : Constant
  Constant5 : Constant
  Send CAN Messages : MotoHawk_lib/CAN Blocks/Send CAN Messages  bus=-2  nam='CAN_1'  msgl=CANTx_AEM_DASH_5  pace=5  labelwires=off
  motohawk_data_read1 : MotoHawk_lib/Data Storage Blocks/motohawk_data_read  source=Lookup By Name  structure=Vector  operation=Read scalar from location by index  sz_vec=4  sz_row=2  sz_col=3  typ=double  nam='InjDC'  checkNull=on  struct_inst_name='MyData'  struct_nam='MyStruct'
  motohawk_data_read2 : MotoHawk_lib/Data Storage Blocks/motohawk_data_read  source=Lookup By Name  structure=Vector  operation=Read scalar from location by index  sz_vec=4  sz_row=2  sz_col=3  typ=double  nam='InjMPW'  checkNull=on  struct_inst_name='MyData'  struct_nam='MyStruct'
  wires:
  Constant/1 -> Send CAN Messages/4
  Constant1/1 -> Send CAN Messages/5
  Constant2/1 -> Send CAN Messages/6
  Constant3/1 -> Send CAN Messages/7
  motohawk_data_read1/1 -> Send CAN Messages/3
  motohawk_data_read2/1 -> Send CAN Messages/1
  Constant4/1 -> motohawk_data_read1/1
  Constant5/1 -> motohawk_data_read2/1
  Data/1 -> Bus Selector/1
  Bus Selector/1 -> Send CAN Messages/2  "<Lambda>"

== system BaseEngineController_LS_128/Foreground/Outputs/AEM Infinity Dash/Dash Message 6 ==
  Data : Inport
  Bus Selector : BusSelector  OutputSignals=Sensors.Raw.LinearSensors.FuelSense,Sensors.RawProcessed.IAT_KeyUp
  Constant : Constant  Value=100
  Constant1 : Constant  Value=100
  Constant{2,4..9} (7 alike) : Constant  Value=0
  Constant3 : Constant  Value=-50
  First Order Low Pass (Tunable) : motohawk_control_primitives_lib/First Order Low Pass (Tunable)  SystemSampleTime=-1  nam='Flex_Filt'  samp_time=-1  group=motohawk_vardec_path(gcb)
  Send CAN Messages : MotoHawk_lib/CAN Blocks/Send CAN Messages  bus=-2  nam='CAN_1'  msgl=CANTx_AEM_DASH_6  pace=5  labelwires=off
  motohawk_data_read : MotoHawk_lib/Data Storage Blocks/motohawk_data_read  source=Lookup By Name  structure=Scalar  operation=Read scalar from location by index  sz_vec=4  sz_row=2  sz_col=3  typ=double  nam='BARO'  checkNull=on  struct_inst_name='MyData'  struct_nam='MyStruct'
  wires:
  Data/1 -> Bus Selector/1
  Constant/1 -> Send CAN Messages/1
  Constant1/1 -> Send CAN Messages/2
  Constant2/1 -> Send CAN Messages/3
  motohawk_data_read/1 -> Send CAN Messages/4
  Bus Selector/1 -> First Order Low Pass (Tunable)/1  "<FuelSense>"
  Bus Selector/2 -> Send CAN Messages/6  "<IAT_KeyUp>"
  Constant3/1 -> Send CAN Messages/7
  Constant4/1 -> Send CAN Messages/8
  Constant5/1 -> Send CAN Messages/9
  Constant6/1 -> Send CAN Messages/10
  Constant7/1 -> Send CAN Messages/11
  Constant8/1 -> Send CAN Messages/12
  Constant9/1 -> Send CAN Messages/13
  First Order Low Pass (Tunable)/1 -> Send CAN Messages/5

== system BaseEngineController_LS_128/Foreground/Outputs/AEM Infinity Dash/Dash Message 7 ==
  Constant : Constant  Value=-50
  Constant1 : Constant  Value=0
  Constant2 : Constant  Value=0
  Constant3 : Constant  Value=0
  Logical Operator : Logic  Operator=OR  Inputs=4  AllPortsSameDT=off  OutDataTypeStr=boolean
  Logical Operator{1..5} (5 alike) : Logic  Operator=OR  AllPortsSameDT=off  OutDataTypeStr=boolean
  Send CAN Messages : MotoHawk_lib/CAN Blocks/Send CAN Messages  bus=-2  nam='CAN_1'  msgl=CANTx_AEM_DASH_7  pace=5  labelwires=off
  motohawk_data_read : MotoHawk_lib/Data Storage Blocks/motohawk_data_read  source=Lookup By Name  structure=Scalar  operation=Read scalar from location by index  sz_vec=4  sz_row=2  sz_col=3  typ=int16  nam='BaseRevLimit'  checkNull=on  struct_inst_name='MyData'  struct_nam='MyStruct'
  motohawk_fault_status1 : MotoHawk_lib/Fault Management Blocks/motohawk_fault_status  source=Lookup By Name  nam='TPS1RangeHigh'  status=Active
  motohawk_fault_status10 : MotoHawk_lib/Fault Management Blocks/motohawk_fault_status  source=Lookup By Name  nam='OilPresRangeLow'  status=Active
  motohawk_fault_status11 : MotoHawk_lib/Fault Management Blocks/motohawk_fault_status  source=Lookup By Name  nam='MAPRangeLow'  status=Active
  motohawk_fault_status12 : MotoHawk_lib/Fault Management Blocks/motohawk_fault_status  source=Lookup By Name  nam='MAPRangeHigh'  status=Active
  motohawk_fault_status13 : MotoHawk_lib/Fault Management Blocks/motohawk_fault_status  source=Lookup By Name  nam='IATRangeLow'  status=Active
  motohawk_fault_status14 : MotoHawk_lib/Fault Management Blocks/motohawk_fault_status  source=Lookup By Name  nam='IATRangeHigh'  status=Active
  motohawk_fault_status2 : MotoHawk_lib/Fault Management Blocks/motohawk_fault_status  source=Lookup By Name  nam='TPS2RangeHigh'  status=Active
  motohawk_fault_status3 : MotoHawk_lib/Fault Management Blocks/motohawk_fault_status  source=Lookup By Name  nam='TPS1RangeLow'  status=Active
  motohawk_fault_status4 : MotoHawk_lib/Fault Management Blocks/motohawk_fault_status  source=Lookup By Name  nam='TPS2RangeLow'  status=Active
  motohawk_fault_status5 : MotoHawk_lib/Fault Management Blocks/motohawk_fault_status  source=Lookup By Name  nam='ECTRangeHigh'  status=Active
  motohawk_fault_status6 : MotoHawk_lib/Fault Management Blocks/motohawk_fault_status  source=Lookup By Name  nam='FuelPresRangeHigh'  status=Active
  motohawk_fault_status7 : MotoHawk_lib/Fault Management Blocks/motohawk_fault_status  source=Lookup By Name  nam='ECTRangeLow'  status=Active
  motohawk_fault_status8 : MotoHawk_lib/Fault Management Blocks/motohawk_fault_status  source=Lookup By Name  nam='FuelPresRangeLow'  status=Active
  motohawk_fault_status9 : MotoHawk_lib/Fault Management Blocks/motohawk_fault_status  source=Lookup By Name  nam='OilPresRangeHigh'  status=Active
  wires:
  Constant/1 -> Send CAN Messages/1
  motohawk_data_read/1 -> Send CAN Messages/2, Send CAN Messages/3
  motohawk_fault_status3/1 -> Logical Operator/1
  motohawk_fault_status1/1 -> Logical Operator/2
  motohawk_fault_status4/1 -> Logical Operator/3
  motohawk_fault_status2/1 -> Logical Operator/4
  Logical Operator/1 -> Send CAN Messages/6
  motohawk_fault_status7/1 -> Logical Operator1/1
  motohawk_fault_status5/1 -> Logical Operator1/2
  Logical Operator1/1 -> Send CAN Messages/7
  motohawk_fault_status8/1 -> Logical Operator2/1
  motohawk_fault_status6/1 -> Logical Operator2/2
  Logical Operator2/1 -> Send CAN Messages/8
  motohawk_fault_status10/1 -> Logical Operator3/1
  motohawk_fault_status9/1 -> Logical Operator3/2
  Logical Operator3/1 -> Send CAN Messages/9
  Constant1/1 -> Send CAN Messages/10
  motohawk_fault_status11/1 -> Logical Operator4/1
  motohawk_fault_status12/1 -> Logical Operator4/2
  Logical Operator4/1 -> Send CAN Messages/11
  motohawk_fault_status13/1 -> Logical Operator5/1
  motohawk_fault_status14/1 -> Logical Operator5/2
  Logical Operator5/1 -> Send CAN Messages/12
  Constant2/1 -> Send CAN Messages/13
  Constant3/1 -> Send CAN Messages/4, Send CAN Messages/5

== system BaseEngineController_LS_128/Foreground/Outputs/AEM Infinity Dash/Dash Message 8 ==
  Constant : Constant  Value=0
  Constant1 : Constant  Value=0
  Constant2 : Constant  Value=0
  Send CAN Messages : MotoHawk_lib/CAN Blocks/Send CAN Messages  bus=-2  nam='CAN_1'  msgl=CANTx_AEM_DASH_8  pace=5  labelwires=off
  wires:
  Constant/1 -> Send CAN Messages/2
  Constant1/1 -> Send CAN Messages/1
  Constant2/1 -> Send CAN Messages/3
